simulink model "TestDebitPapillonNew"  (R2024b)
settings: Solver=VariableStepAuto  StartTime=0.0  StopTime=10.0  RelTol=1e-3
undefined symbols (not defined in the file): AirIntakeAirFlowTest, AirIntakeTemperatureTest, AirIntakeTimeTest, gam, Pamb, PcolPapTest, PRcrit, Rair, SectionPapTest, Tamb, TempsPapTest
settings Model: Creator=a030141  LastModifiedBy=ramse
settings DebuggingCC: UnderspecifiedInitializationDetection=Classic  MergeDetectMultiDrivingBlocksExec=none
settings ModelReferenceCC: PropagateSignalLabelsOutOfModel=off

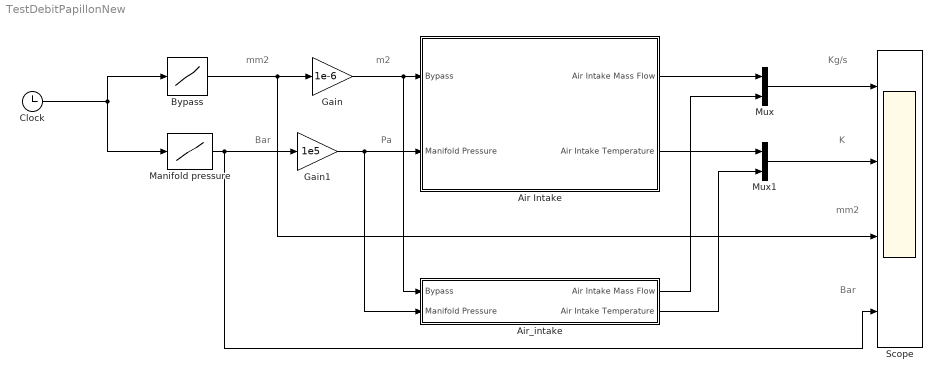
== system TestDebitPapillonNew ==
  note: m2
  note: mm2
  note: Pa
  note: mm2
  note: K
  note: Kg/s
  note: Bar
  note: Bar
  Air Intake : Subsystem
  Air_intake : Subsystem
  Bypass : Lookup  InputValues=TempsPapTest  Table=SectionPapTest
  Clock : Clock
  Gain : Gain  Gain=1e-6  SaturateOnIntegerOverflow=on  OutDataTypeStr=Inherit: Same as input  ParamDataTypeStr=Inherit: Same as input
  Gain1 : Gain  Gain=1e5  SaturateOnIntegerOverflow=on  OutDataTypeStr=Inherit: Same as input  ParamDataTypeStr=Inherit: Same as input
  Manifold pressure : Lookup  InputValues=TempsPapTest  Table=PcolPapTest
  Mux : Mux  Inputs=2
  Mux1 : Mux  Inputs=2
  Scope : Scope  NumInputPorts=4
  wires:
  Manifold pressure/1 -> Gain1/1, Scope/4
  Clock/1 -> Bypass/1, Manifold pressure/1
  Bypass/1 -> Gain/1, Scope/3
  Gain1/1 -> Air_intake/2(Manifold Pressure), Air Intake/2(Manifold Pressure)
  Mux/1 -> Scope/1
  Mux1/1 -> Scope/2
  Air Intake/1(Air Intake Mass Flow) -> Mux/1
  Air Intake/2(Air Intake Temperature) -> Mux1/1
  Gain/1 -> Air_intake/1(Bypass), Air Intake/1(Bypass)
  Air_intake/1(Air Intake Mass Flow) -> Mux/2
  Air_intake/2(Air Intake Temperature) -> Mux1/2

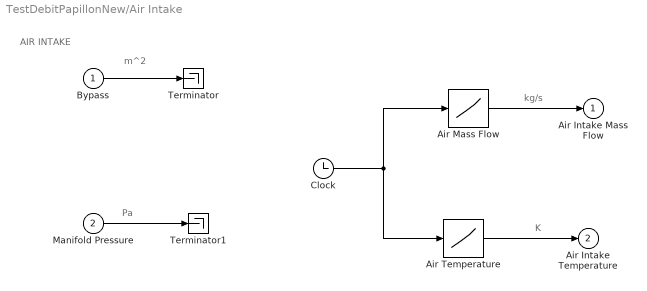
== system TestDebitPapillonNew/Air Intake ==
  note: AIR INTAKE
  note: m^2
  note: kg/s
  note: Pa
  note: K
  Bypass : Inport
  Manifold Pressure : Inport  Port=2
  Air Mass Flow : Lookup  InputValues=AirIntakeTimeTest  Table=AirIntakeAirFlowTest
  Air Temperature : Lookup  InputValues=AirIntakeTimeTest  Table=AirIntakeTemperatureTest
  Clock : Clock
  Terminator : Terminator
  Terminator1 : Terminator
  Air Intake Mass Flow : Outport
  Air Intake Temperature : Outport  Port=2
  wires:
  Air Mass Flow/1 -> Air Intake Mass Flow/1
  Manifold Pressure/1 -> Terminator1/1
  Bypass/1 -> Terminator/1
  Air Temperature/1 -> Air Intake Temperature/1
  Clock/1 -> Air Mass Flow/1, Air Temperature/1

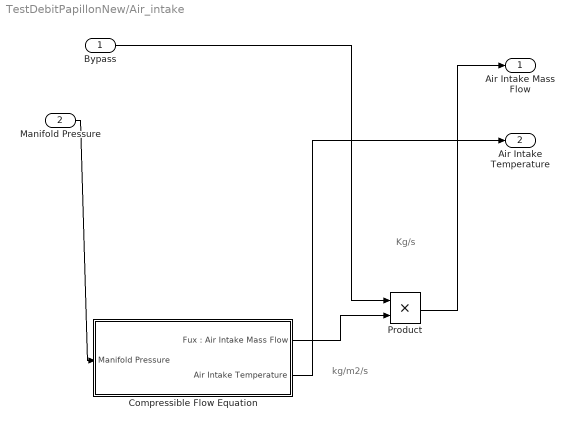
== system TestDebitPapillonNew/Air_intake ==
  note: Kg/s
  note: kg/m2/s
  Bypass : Inport
  Manifold Pressure : Inport  Port=2
  Compressible Flow Equation : Subsystem
  Product : Product
  Air Intake Mass Flow : Outport
  Air Intake Temperature : Outport  Port=2
  wires:
  Compressible Flow Equation/2(Air Intake Temperature) -> Air Intake Temperature/1
  Compressible Flow Equation/1("Fux : Air Intake Mass Flow") -> Product/2
  Manifold Pressure/1 -> Compressible Flow Equation/1(Manifold Pressure)
  Product/1 -> Air Intake Mass Flow/1
  Bypass/1 -> Product/1

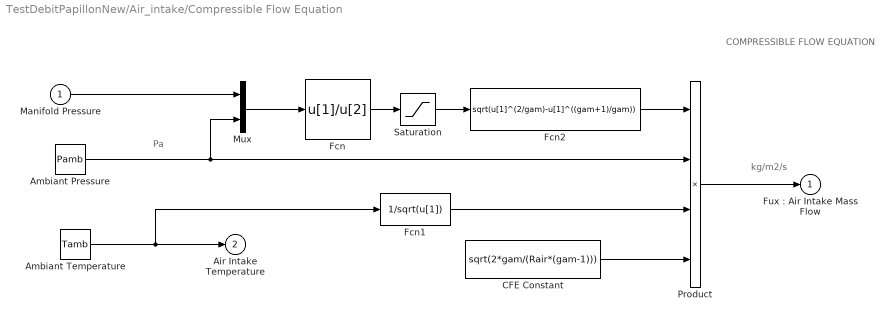
== system TestDebitPapillonNew/Air_intake/Compressible Flow Equation ==
  note: COMPRESSIBLE FLOW EQUATION
  note: Pa
  note: kg/m2/s
  Manifold Pressure : Inport
  Ambiant Pressure : Constant  Value=Pamb
  Ambiant Temperature : Constant  Value=Tamb
  "CFE Constant " : Constant  Value=sqrt(2*gam/(Rair*(gam-1)))
  Fcn : Fcn  Expr=u[1]/u[2]
  Fcn1 : Fcn  Expr=1/sqrt(u[1])
  Fcn2 : Fcn  Expr=sqrt(u[1]^(2/gam)-u[1]^((gam+1)/gam))
  Mux : Mux  Inputs=2
  Product : Product  Inputs=4  InputSameDT=on  SaturateOnIntegerOverflow=on  OutDataTypeStr=Inherit: Same as first input
  Saturation : Saturate  UpperLimit=1  LowerLimit=PRcrit
  "Fux : Air Intake Mass Flow" : Outport
  Air Intake Temperature : Outport  Port=2
  wires:
  Ambiant Pressure/1 -> Product/2, Mux/2
  Product/1 -> "Fux : Air Intake Mass Flow"/1
  "CFE Constant "/1 -> Product/4
  Fcn2/1 -> Product/1
  Saturation/1 -> Fcn2/1
  Fcn1/1 -> Product/3
  Fcn/1 -> Saturation/1
  Mux/1 -> Fcn/1
  Manifold Pressure/1 -> Mux/1
  Ambiant Temperature/1 -> Fcn1/1, Air Intake Temperature/1
